simulink model "model"  (R2022a)
settings: Solver=VariableStepAuto  StartTime=0.0  StopTime=0.1  MaxStep=0.0001  RelTol=1e-3
values from neighbouring files (symbols this model uses):
  betta = Mp/wnom    (= 0.600343053173)    [config.m]
  ELMEX = 0    [config.m]    (also in tasks.m = 1)
  J = J1+J2    (= 0.01)    [config.m]
  Km = u_zad/Mnom    (= 1.39664804469)    [config.m]
  Kp = Te/(2*Tpr*Kpr*Km*betta)    (= 0.393574971429)    [config.m]
  Kpr = 10    [config.m]
  Te = 3.3/1000    (= 0.0033)    [config.m]
  Ti = Te    (= 0.0033)    [config.m]
  Tmu = Tpr    (= 0.0005)    [config.m]
  Tpr = 0.5/1000    (= 0.0005)    [config.m]
undefined symbols (not defined in the file or in its folder): Mzad
settings Model: Creator=Vvlad  LastModifiedBy=Vvlad

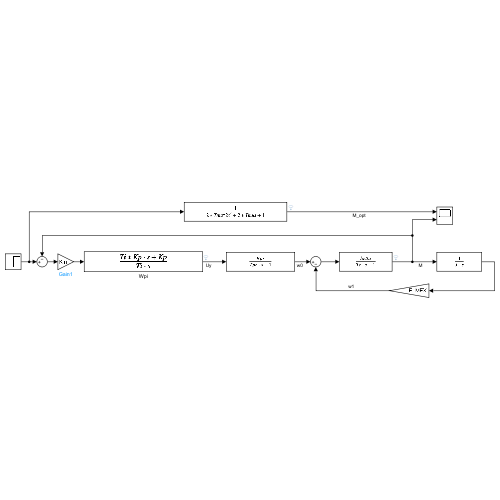
[thumbnail: Simulink's stored preview of the top-level diagram]
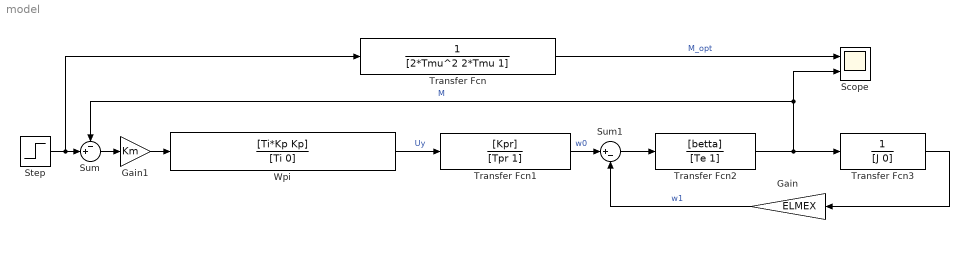
== system model ==
  Gain : Gain  Gain=ELMEX
  Gain1 : Gain  Gain=Km
  Scope : Scope  NumInputPorts=2
  Step : Step  Time=0  After=Mzad  SampleTime=0
  Sum : Sum  Inputs=-+|
  Sum1 : Sum  Inputs=|+-
  Transfer Fcn : TransferFcn  Denominator=[2*Tmu^2 2*Tmu 1]
  Transfer Fcn1 : TransferFcn  Numerator=[Kpr]  Denominator=[Tpr 1]
  Transfer Fcn2 : TransferFcn  Numerator=[betta]  Denominator=[Te 1]
  Transfer Fcn3 : TransferFcn  Denominator=[J 0]
  Wpi : TransferFcn  Numerator=[Ti*Kp Kp]  Denominator=[Ti 0]
  wires:
  Transfer Fcn/1 -> Scope/1  "M_opt"
  Sum/1 -> Gain1/1
  Transfer Fcn2/1 -> Sum/1, Scope/2, Transfer Fcn3/1  "M"
  Transfer Fcn1/1 -> Sum1/1  "w0"
  Wpi/1 -> Transfer Fcn1/1  "Uy"
  Step/1 -> Transfer Fcn/1, Sum/2
  Transfer Fcn3/1 -> Gain/1
  Sum1/1 -> Transfer Fcn2/1
  Gain/1 -> Sum1/2  "w1"
  Gain1/1 -> Wpi/1
